simulink subsystem "Electromechanical_SubSystem"  (R2020b)
settings: Solver=VariableStepAuto  StartTime=0.0  StopTime=10.0  RelTol=1e-3
undefined symbols (not defined in the file or in its folder): Fv1, Ts, ua2tau, x0
settings Model: Creator=umberto  LastModifiedBy=umberto

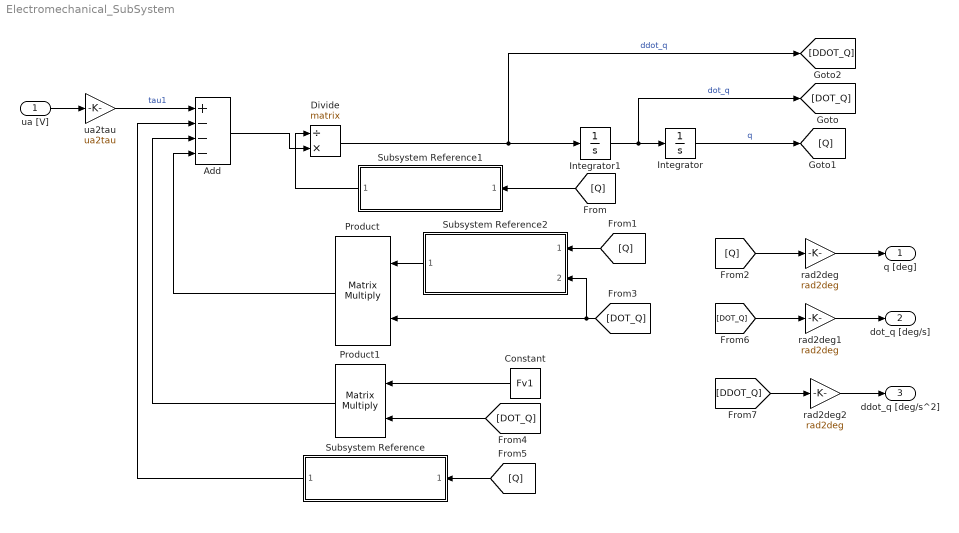
== system Electromechanical_SubSystem ==
  ua [V] : Inport
  Add : Sum  Inputs=+---
  Constant : Constant  Value=Fv1  SampleTime=Ts
  Divide : Product  Inputs=/*  Multiplication=Matrix(*)
  Integrator : Integrator  InitialCondition=x0(1:2)
  Integrator1 : Integrator  InitialCondition=x0(3:end)
  Product : Product  Multiplication=Matrix(*)
  Product1 : Product  Multiplication=Matrix(*)
  Subsystem Reference : Subsystem  ReferencedSubsystem=gq_SubSystem
  Subsystem Reference1 : Subsystem  ReferencedSubsystem=Mq_SubSystem
  Subsystem Reference2 : Subsystem  ReferencedSubsystem=Cqdot_q_SubSystem
  rad2deg : Gain  Gain=rad2deg
  rad2deg1 : Gain  Gain=rad2deg
  rad2deg2 : Gain  Gain=rad2deg
  ua2tau : Gain  Gain=ua2tau
  q [deg] : Outport
  dot_q [deg/s] : Outport  Port=2
  ddot_q [deg/s^2] : Outport  Port=3
  wires:
  ua [V]/1 -> ua2tau/1
  ua2tau/1 -> Add/1  "tau1"
  rad2deg/1 -> q [deg]/1
  rad2deg1/1 -> dot_q [deg/s]/1
  rad2deg2/1 -> ddot_q [deg/s^2]/1
  Subsystem Reference/1 -> Add/2
  Subsystem Reference2/1 -> Product/1
  [Q] -> Subsystem Reference1/1
  [Q] -> Subsystem Reference2/1
  [Q] -> rad2deg/1
  [DOT_Q] -> Subsystem Reference2/2, Product/2
  Product/1 -> Add/4
  Constant/1 -> Product1/1
  [DOT_Q] -> Product1/2
  [Q] -> Subsystem Reference/1
  Product1/1 -> Add/3
  Add/1 -> Divide/2
  Subsystem Reference1/1 -> Divide/1
  Divide/1 -> [DDOT_Q], Integrator1/1  "ddot_q"
  Integrator/1 -> [Q]  "q"
  Integrator1/1 -> [DOT_Q], Integrator/1  "dot_q"
  [DDOT_Q] -> rad2deg2/1
  [DOT_Q] -> rad2deg1/1
